simulink model "target_groundpass_test"  (R2018b)
settings: Solver=VariableStepAuto  StartTime=0.0  StopTime=86400  RelTol=1e-3
undefined symbols (not defined in the file): fswParams, simParams
libraries: simulink_extras x1, sgp4_lib_fsw x1, time_coord_rotations_lib x1, target_groundpass_lib x1
settings Model: Creator=Taylor  LastModifiedBy=Taylor

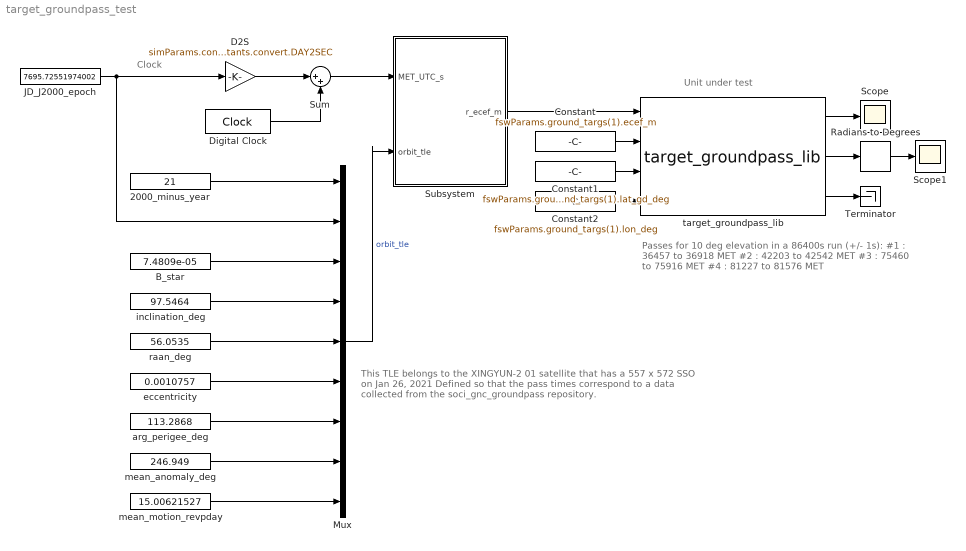
== system target_groundpass_test ==
  note: Clock
  note: Passes for 10 deg elevation in a 86400s run (+/- 1s):
      | #1 : 36457 to 36918 MET
      | #2 : 42203 to 42542 MET
      | #3 : 75460 to 75916 MET
      | #4 : 81227 to 81576 MET
  note: This TLE belongs to the XINGYUN-2 01 satellite
      | that has a 557 x 572 SSO on Jan 26, 2021
      |
      | Defined so that the pass times correspond to
      | a data collected from the
      | soci_gnc_groundpass
      | repository.
  note: Unit under test
  2000_minus_year : Constant  Value=21
  B_star : Constant  Value=7.4809e-05
  Constant : Constant  Value=fswParams.ground_targs(1).ecef_m
  Constant1 : Constant  Value=fswParams.ground_targs(1).lat_gd_deg
  Constant2 : Constant  Value=fswParams.ground_targs(1).lon_deg
  D2S : Gain  Gain=simParams.constants.convert.DAY2SEC
  Digital Clock : DigitalClock  SampleTime=simParams.sample_time_s
  JD_J2000_epoch : Constant  Value=7695.72551974002
  Mux : Mux  Inputs=9
  Radians to Degrees : simulink_extras/Transformations/Radians to Degrees
  Scope : Scope
  Scope1 : Scope
  Subsystem : Subsystem
  Sum : Sum  Inputs=|++
  Terminator : Terminator
  arg_perigee_deg : Constant  Value=113.2868
  eccentricity : Constant  Value=0.0010757
  inclination_deg : Constant  Value=97.5464
  mean_anomaly_deg : Constant  Value=246.949
  mean_motion_revpday : Constant  Value=15.00621527
  raan_deg : Constant  Value=56.0535
  target_groundpass_lib : target_groundpass_lib/target_groundpass_lib  id=1
  wires:
  Mux/1 -> Subsystem/2(orbit_tle)  "orbit_tle"
  Subsystem/1(r_ecef_m) -> target_groundpass_lib/1
  Constant/1 -> target_groundpass_lib/2
  Constant1/1 -> target_groundpass_lib/3
  Constant2/1 -> target_groundpass_lib/4
  target_groundpass_lib/1 -> Scope/1
  target_groundpass_lib/2 -> Radians to Degrees/1
  target_groundpass_lib/3 -> Terminator/1
  2000_minus_year/1 -> Mux/1
  inclination_deg/1 -> Mux/4
  eccentricity/1 -> Mux/6
  JD_J2000_epoch/1 -> Mux/2, D2S/1
  B_star/1 -> Mux/3
  raan_deg/1 -> Mux/5
  arg_perigee_deg/1 -> Mux/7
  mean_anomaly_deg/1 -> Mux/8
  mean_motion_revpday/1 -> Mux/9
  Radians to Degrees/1 -> Scope1/1
  D2S/1 -> Sum/1
  Digital Clock/1 -> Sum/2
  Sum/1 -> Subsystem/1(MET_UTC_s)

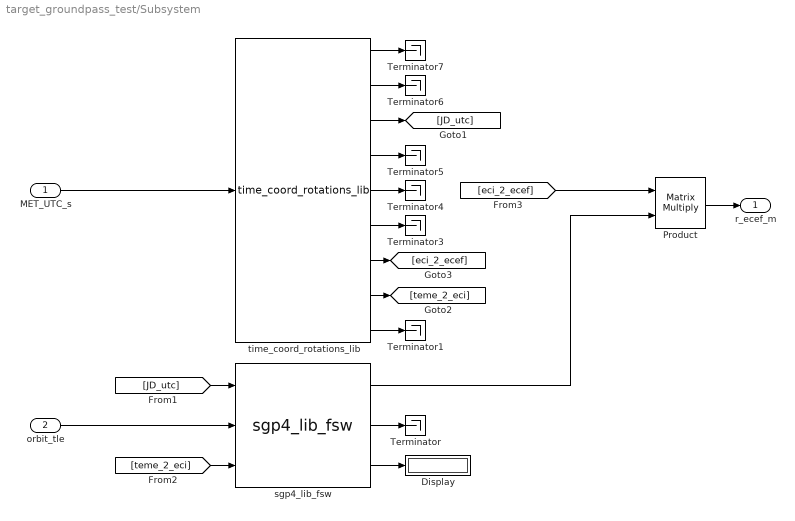
== system target_groundpass_test/Subsystem ==
  MET_UTC_s : Inport
  orbit_tle : Inport  Port=2
  Display : Display
  Product : Product  Multiplication=Matrix(*)
  Terminator{,1,3..7} (7 alike) : Terminator
  sgp4_lib_fsw : sgp4_lib_fsw/sgp4_lib_fsw  SystemSampleTime=-1
  "time_coord_rotations_lib " : time_coord_rotations_lib/time_coord_rotations_lib    SystemSampleTime=-1
  r_ecef_m : Outport
  wires:
  MET_UTC_s/1 -> "time_coord_rotations_lib "/1
  "time_coord_rotations_lib "/1 -> Terminator7/1
  [teme_2_eci] -> sgp4_lib_fsw/3
  "time_coord_rotations_lib "/4 -> Terminator5/1
  "time_coord_rotations_lib "/5 -> Terminator4/1
  "time_coord_rotations_lib "/6 -> Terminator3/1
  sgp4_lib_fsw/2 -> Terminator/1
  "time_coord_rotations_lib "/9 -> Terminator1/1
  [JD_utc] -> sgp4_lib_fsw/1
  "time_coord_rotations_lib "/7 -> [eci_2_ecef]
  "time_coord_rotations_lib "/2 -> Terminator6/1
  sgp4_lib_fsw/3 -> Display/1
  "time_coord_rotations_lib "/3 -> [JD_utc]
  "time_coord_rotations_lib "/8 -> [teme_2_eci]
  orbit_tle/1 -> sgp4_lib_fsw/2
  [eci_2_ecef] -> Product/1
  sgp4_lib_fsw/1 -> Product/2
  Product/1 -> r_ecef_m/1
